simulink model "verification"  (R2012b)
settings: Solver=FixedStepDiscrete  StartTime=0.0  StopTime=10.0  FixedStep=0.1  RelTol=1e-3
undefined symbols (not defined in the file): sldvsubsys
libraries: sldvlib x21
settings Model: Creator=z2akhtar  LastModifiedBy=z2akhtar
settings ConfigComp: Description=Design Verifier Custom Configuration Component  DVMode=PropertyProving  DVMaxProcessTime=1800  DVMaxTestCaseSteps=500  DVTestSuiteOptimization=CombinedObjectives (Nonlinear Extended)  DVProvingStrategy=ProveWithViolationDetection  DVMaxViolationSteps=10

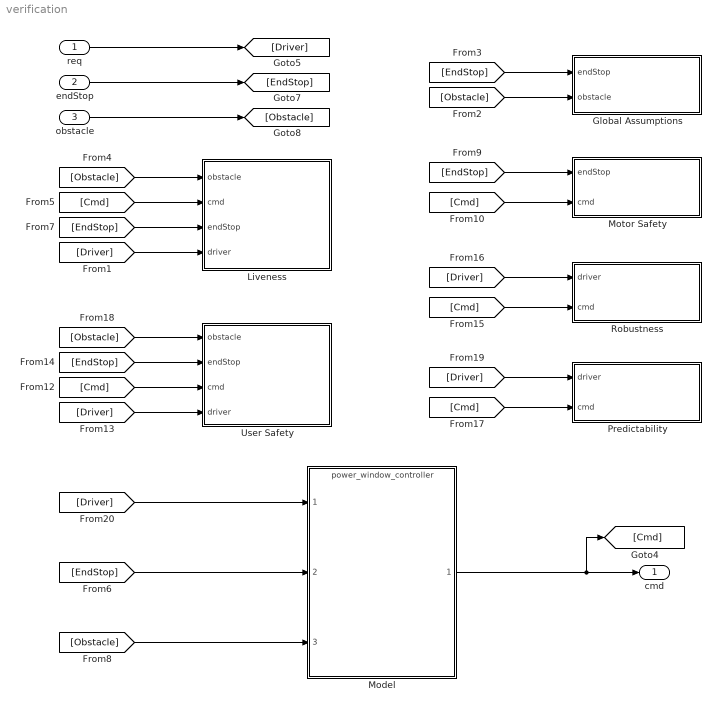
== system verification ==
  req : Inport  OutDataTypeStr=double
  endStop : Inport  Port=2  OutDataTypeStr=boolean
  obstacle : Inport  Port=3  OutDataTypeStr=boolean
  Global Assumptions : Subsystem  Tag=VerificationSubsystem  DisableCoverage=on  LoadFcn=sldvsubsys('check')  TreatAsAtomicUnit=on  SimViewingDevice=on  mask(VerificationSubsystem){}
      mask init:
      | sldvsubsys('maskInit');
      settings: CopyFcn=sldvsubsys('copy');  OpenFcn=open_system(gcb,'force');
      settings: PreSaveFcn=|
      | set_param(gcb,'SimViewingDevice','on');
      | sldvsubsys('check');
      mask Help: helpview(fullfile(docroot,'toolbox','sldv','sldv.map'),'verificationsubsystem')
      mask Display: image(imread('sldvicon_versubsys.png','BackGroundColor',[1 1 1]),'center');
  Liveness : Subsystem  Tag=VerificationSubsystem  DisableCoverage=on  LoadFcn=sldvsubsys('check')  TreatAsAtomicUnit=on  SimViewingDevice=on  mask(VerificationSubsystem){}
      mask init:
      | sldvsubsys('maskInit');
      settings: CopyFcn=sldvsubsys('copy');  OpenFcn=open_system(gcb,'force');
      settings: PreSaveFcn=|
      | set_param(gcb,'SimViewingDevice','on');
      | sldvsubsys('check');
      mask Help: helpview(fullfile(docroot,'toolbox','sldv','sldv.map'),'verificationsubsystem')
      mask Display: image(imread('sldvicon_versubsys.png','BackGroundColor',[1 1 1]),'center');
  Model : ModelReference  ModelNameDialog=power_window_controller  SimulationMode=Normal  ModelReferenceVersion=1.36  CopyOfModelName=power_window_controller  DefaultDataLogging=on
  Motor Safety : Subsystem  Tag=VerificationSubsystem  DisableCoverage=on  LoadFcn=sldvsubsys('check')  TreatAsAtomicUnit=on  SimViewingDevice=on  mask(VerificationSubsystem){}
      mask init:
      | sldvsubsys('maskInit');
      settings: CopyFcn=sldvsubsys('copy');  OpenFcn=open_system(gcb,'force');
      settings: PreSaveFcn=|
      | set_param(gcb,'SimViewingDevice','on');
      | sldvsubsys('check');
      mask Help: helpview(fullfile(docroot,'toolbox','sldv','sldv.map'),'verificationsubsystem')
      mask Display: image(imread('sldvicon_versubsys.png','BackGroundColor',[1 1 1]),'center');
  Predictability : Subsystem  Tag=VerificationSubsystem  DisableCoverage=on  LoadFcn=sldvsubsys('check')  TreatAsAtomicUnit=on  SimViewingDevice=on  mask(VerificationSubsystem){}
      mask init:
      | sldvsubsys('maskInit');
      settings: CopyFcn=sldvsubsys('copy');  OpenFcn=open_system(gcb,'force');
      settings: PreSaveFcn=|
      | set_param(gcb,'SimViewingDevice','on');
      | sldvsubsys('check');
      mask Help: helpview(fullfile(docroot,'toolbox','sldv','sldv.map'),'verificationsubsystem')
      mask Display: image(imread('sldvicon_versubsys.png','BackGroundColor',[1 1 1]),'center');
  Robustness : Subsystem  Tag=VerificationSubsystem  DisableCoverage=on  LoadFcn=sldvsubsys('check')  TreatAsAtomicUnit=on  SimViewingDevice=on  mask(VerificationSubsystem){}
      mask init:
      | sldvsubsys('maskInit');
      settings: CopyFcn=sldvsubsys('copy');  OpenFcn=open_system(gcb,'force');
      settings: PreSaveFcn=|
      | set_param(gcb,'SimViewingDevice','on');
      | sldvsubsys('check');
      mask Help: helpview(fullfile(docroot,'toolbox','sldv','sldv.map'),'verificationsubsystem')
      mask Display: image(imread('sldvicon_versubsys.png','BackGroundColor',[1 1 1]),'center');
  User Safety : Subsystem  Tag=VerificationSubsystem  DisableCoverage=on  LoadFcn=sldvsubsys('check')  TreatAsAtomicUnit=on  SimViewingDevice=on  mask(VerificationSubsystem){}
      mask init:
      | sldvsubsys('maskInit');
      settings: CopyFcn=sldvsubsys('copy');  OpenFcn=open_system(gcb,'force');
      settings: PreSaveFcn=|
      | set_param(gcb,'SimViewingDevice','on');
      | sldvsubsys('check');
      mask Help: helpview(fullfile(docroot,'toolbox','sldv','sldv.map'),'verificationsubsystem')
      mask Display: image(imread('sldvicon_versubsys.png','BackGroundColor',[1 1 1]),'center');
  cmd : Outport
  wires:
  Model/1 -> [Cmd], cmd/1
  req/1 -> [Driver]
  endStop/1 -> [EndStop]
  obstacle/1 -> [Obstacle]
  [Obstacle] -> Global Assumptions/2(obstacle)
  [EndStop] -> Global Assumptions/1(endStop)
  [EndStop] -> Motor Safety/1(endStop)
  [Cmd] -> Motor Safety/2(cmd)
  [EndStop] -> User Safety/2(endStop)
  [Cmd] -> User Safety/3(cmd)
  [Driver] -> User Safety/4(driver)
  [Driver] -> Model/1
  [EndStop] -> Model/2
  [Obstacle] -> Model/3
  [Cmd] -> Robustness/2(cmd)
  [Driver] -> Robustness/1(driver)
  [Obstacle] -> User Safety/1(obstacle)
  [Obstacle] -> Liveness/1(obstacle)
  [Cmd] -> Liveness/2(cmd)
  [EndStop] -> Liveness/3(endStop)
  [Driver] -> Liveness/4(driver)
  [Cmd] -> Predictability/2(cmd)
  [Driver] -> Predictability/1(driver)

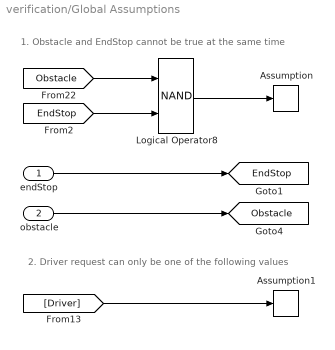
== system verification/Global Assumptions ==
  note: 1. Obstacle and EndStop cannot be true at the same time
  note: 2. Driver request can only be one of the following values
  endStop : Inport
  obstacle : Inport  Port=2
  Assumption : sldvlib/Objectives and Constraints/Assumption  enabled=on  customAVTBlockType=Assumption  intervals=true  initial=off  dispValues=on  outEnabled=off
      settings: AttributesFormatString=%<intervals>
  Assumption1 : sldvlib/Objectives and Constraints/Assumption  enabled=on  customAVTBlockType=Assumption  intervals={0,1,2,3,4}  initial=off  dispValues=on  outEnabled=off
      settings: AttributesFormatString=%<intervals>
  Logical Operator8 : Logic  Operator=NAND  AllPortsSameDT=off  OutDataTypeStr=boolean
  tag scope: EndStop=global, Obstacle=global
  wires:
  [Obstacle] -> Logical Operator8/1
  Logical Operator8/1 -> Assumption/1
  [EndStop] -> Logical Operator8/2
  endStop/1 -> [EndStop]
  obstacle/1 -> [Obstacle]
  [Driver] -> Assumption1/1

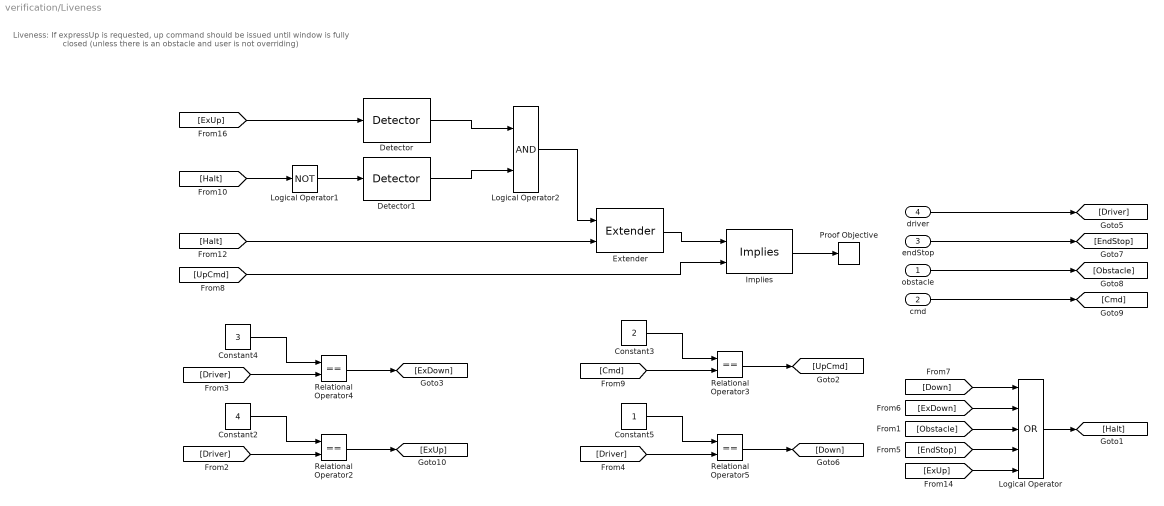
== system verification/Liveness ==
  note: Liveness:
      | If expressUp is requested, up command should be issued until window is fully closed (unless there is an obstacle and user is not overriding)
  obstacle : Inport  OutDataTypeStr=boolean
  cmd : Inport  Port=2
  endStop : Inport  Port=3  OutDataTypeStr=boolean
  driver : Inport  Port=4  OutDataTypeStr=double
  Constant2 : Constant  Value=4  SampleTime=Inf
  Constant3 : Constant  Value=2  SampleTime=Inf
  Constant4 : Constant  Value=3  SampleTime=Inf
  Constant5 : Constant  SampleTime=Inf
  Detector : sldvlib/Temporal Operators/Detector  reset=off  typ=Delayed Fixed Duration  in_hold=3  delay=0  out_hold=2
  Detector1 : sldvlib/Temporal Operators/Detector  reset=off  typ=Delayed Fixed Duration  in_hold=4  delay=0  out_hold=1
  Extender : sldvlib/Temporal Operators/Extender  reset=on  ext_type=Infinite  out_hold=3
  Implies : sldvlib/Verification Utilities/Implies
  Logical Operator : Logic  Operator=OR  Inputs=5  AllPortsSameDT=off  OutDataTypeStr=boolean
  Logical Operator1 : Logic  Operator=NOT  AllPortsSameDT=off  OutDataTypeStr=boolean
  Logical Operator2 : Logic  AllPortsSameDT=off  OutDataTypeStr=boolean
  Proof Objective : sldvlib/Objectives and Constraints/Proof Objective  enabled=on  customAVTBlockType=Proof Objective  intervals=true  dispValues=on  outEnabled=off  enableStopSim=off
      settings: AttributesFormatString=%<intervals>
  Relational Operator{2..5} (4 alike) : RelationalOperator  Operator===  OutDataTypeStr=boolean
  wires:
  Implies/1 -> Proof Objective/1
  [Driver] -> Relational Operator2/2
  Constant2/1 -> Relational Operator2/1
  Relational Operator2/1 -> [ExUp]
  [ExUp] -> Detector/1
  [Cmd] -> Relational Operator3/2
  Constant3/1 -> Relational Operator3/1
  Relational Operator3/1 -> [UpCmd]
  driver/1 -> [Driver]
  endStop/1 -> [EndStop]
  obstacle/1 -> [Obstacle]
  [Driver] -> Relational Operator4/2
  Constant4/1 -> Relational Operator4/1
  Relational Operator4/1 -> [ExDown]
  [Driver] -> Relational Operator5/2
  Constant5/1 -> Relational Operator5/1
  Relational Operator5/1 -> [Down]
  Logical Operator/1 -> [Halt]
  [Down] -> Logical Operator/1
  [ExDown] -> Logical Operator/2
  [Obstacle] -> Logical Operator/3
  [EndStop] -> Logical Operator/4
  cmd/1 -> [Cmd]
  [Halt] -> Logical Operator1/1
  Logical Operator2/1 -> Extender/1
  [Halt] -> Extender/2
  [UpCmd] -> Implies/2
  Extender/1 -> Implies/1
  Detector/1 -> Logical Operator2/1
  Logical Operator1/1 -> Detector1/1
  Detector1/1 -> Logical Operator2/2
  [ExUp] -> Logical Operator/5

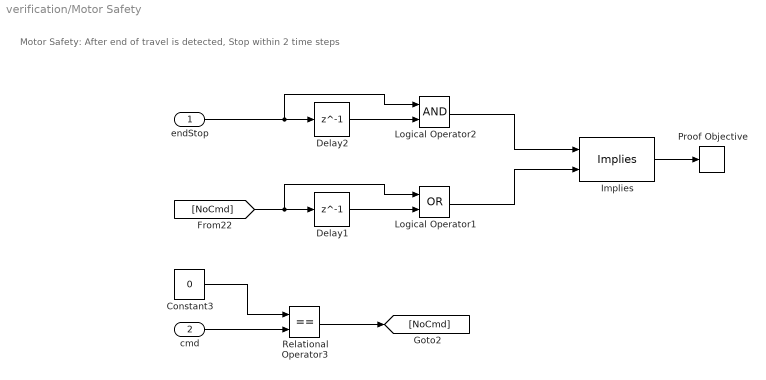
== system verification/Motor Safety ==
  note: Motor Safety:
      | After end of travel is detected, Stop within 2 time steps
  endStop : Inport
  cmd : Inport  Port=2
  Constant3 : Constant  Value=0  SampleTime=Inf
  Delay1 : Delay  DelayLength=1  InitialCondition=0
  Delay2 : Delay  DelayLength=1  InitialCondition=0
  Implies : sldvlib/Verification Utilities/Implies
  Logical Operator1 : Logic  Operator=OR  AllPortsSameDT=off  OutDataTypeStr=boolean
  Logical Operator2 : Logic  AllPortsSameDT=off  OutDataTypeStr=boolean
  Proof Objective : sldvlib/Objectives and Constraints/Proof Objective  enabled=off  customAVTBlockType=Proof Objective  intervals=true  dispValues=on  outEnabled=off  enableStopSim=off
      settings: AttributesFormatString=%<intervals>
  Relational Operator3 : RelationalOperator  Operator===  OutDataTypeStr=boolean
  wires:
  Implies/1 -> Proof Objective/1
  Delay1/1 -> Logical Operator1/2
  [NoCmd] -> Delay1/1, Logical Operator1/1
  cmd/1 -> Relational Operator3/2
  Constant3/1 -> Relational Operator3/1
  Relational Operator3/1 -> [NoCmd]
  Delay2/1 -> Logical Operator2/2
  endStop/1 -> Delay2/1, Logical Operator2/1
  Logical Operator2/1 -> Implies/1
  Logical Operator1/1 -> Implies/2

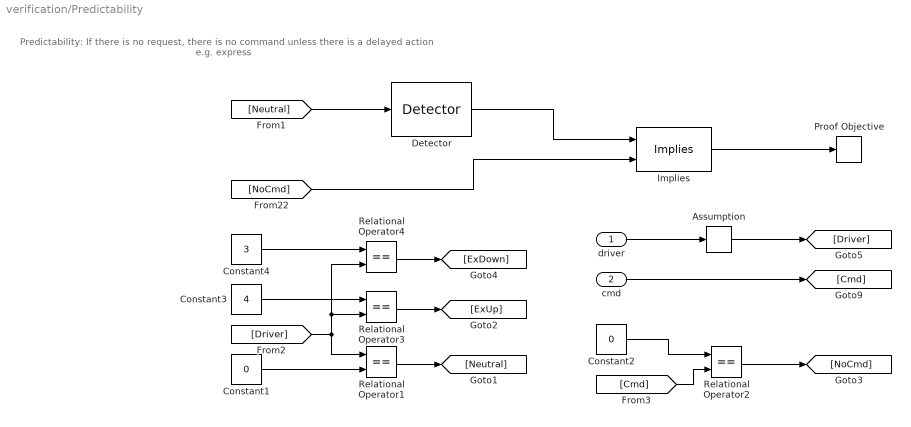
== system verification/Predictability ==
  note: Predictability:
      | If there is no request, there is no command unless there is a delayed action e.g. express
  driver : Inport  OutDataTypeStr=double
  cmd : Inport  Port=2
  Assumption : sldvlib/Objectives and Constraints/Assumption  enabled=on  customAVTBlockType=Assumption  intervals={0,1,2}  initial=off  dispValues=on  outEnabled=on
      settings: AttributesFormatString=%<intervals>
  Constant1 : Constant  Value=0  SampleTime=Inf
  Constant2 : Constant  Value=0  SampleTime=Inf
  Constant3 : Constant  Value=4  SampleTime=Inf
  Constant4 : Constant  Value=3  SampleTime=Inf
  Detector : sldvlib/Temporal Operators/Detector  reset=off  typ=Synchronized  in_hold=3  delay=0  out_hold=5
  Implies : sldvlib/Verification Utilities/Implies
  Proof Objective : sldvlib/Objectives and Constraints/Proof Objective  enabled=on  customAVTBlockType=Proof Objective  intervals=true  dispValues=on  outEnabled=off  enableStopSim=off
      settings: AttributesFormatString=%<intervals>
  Relational Operator{1..4} (4 alike) : RelationalOperator  Operator===  OutDataTypeStr=boolean
  wires:
  Implies/1 -> Proof Objective/1
  [Driver] -> Relational Operator4/2, Relational Operator3/2, Relational Operator1/1
  Relational Operator3/1 -> [ExUp]
  Constant1/1 -> Relational Operator1/2
  Constant3/1 -> Relational Operator3/1
  Relational Operator1/1 -> [Neutral]
  [Neutral] -> Detector/1
  Relational Operator2/1 -> [NoCmd]
  cmd/1 -> [Cmd]
  Constant4/1 -> Relational Operator4/1
  Relational Operator4/1 -> [ExDown]
  driver/1 -> Assumption/1
  Assumption/1 -> [Driver]
  Detector/1 -> Implies/1
  [Cmd] -> Relational Operator2/2
  Constant2/1 -> Relational Operator2/1
  [NoCmd] -> Implies/2

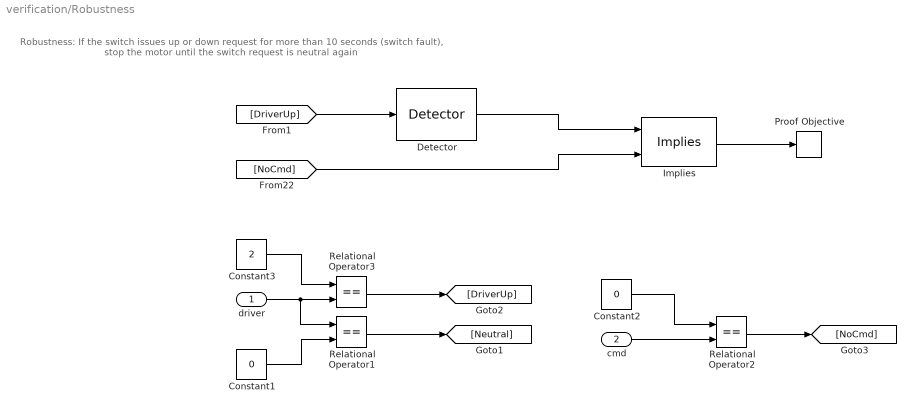
== system verification/Robustness ==
  note: Robustness:
      | If the switch issues up or down request for more than 10 seconds (switch fault), stop the motor until the switch request is neutral again
  driver : Inport
  cmd : Inport  Port=2
  Constant1 : Constant  Value=0  SampleTime=Inf
  Constant2 : Constant  Value=0  SampleTime=Inf
  Constant3 : Constant  Value=2  SampleTime=Inf
  Detector : sldvlib/Temporal Operators/Detector  reset=off  typ=Delayed Fixed Duration  in_hold=100  delay=0  out_hold=5
  Implies : sldvlib/Verification Utilities/Implies
  Proof Objective : sldvlib/Objectives and Constraints/Proof Objective  enabled=off  customAVTBlockType=Proof Objective  intervals=true  dispValues=on  outEnabled=off  enableStopSim=off
      settings: AttributesFormatString=%<intervals>
  Relational Operator1 : RelationalOperator  Operator===  OutDataTypeStr=boolean
  Relational Operator2 : RelationalOperator  Operator===  OutDataTypeStr=boolean
  Relational Operator3 : RelationalOperator  Operator===  OutDataTypeStr=boolean
  wires:
  Implies/1 -> Proof Objective/1
  driver/1 -> Relational Operator1/1, Relational Operator3/2
  Relational Operator3/1 -> [DriverUp]
  [NoCmd] -> Implies/2
  Constant1/1 -> Relational Operator1/2
  Constant3/1 -> Relational Operator3/1
  Relational Operator1/1 -> [Neutral]
  [DriverUp] -> Detector/1
  Detector/1 -> Implies/1
  cmd/1 -> Relational Operator2/2
  Constant2/1 -> Relational Operator2/1
  Relational Operator2/1 -> [NoCmd]

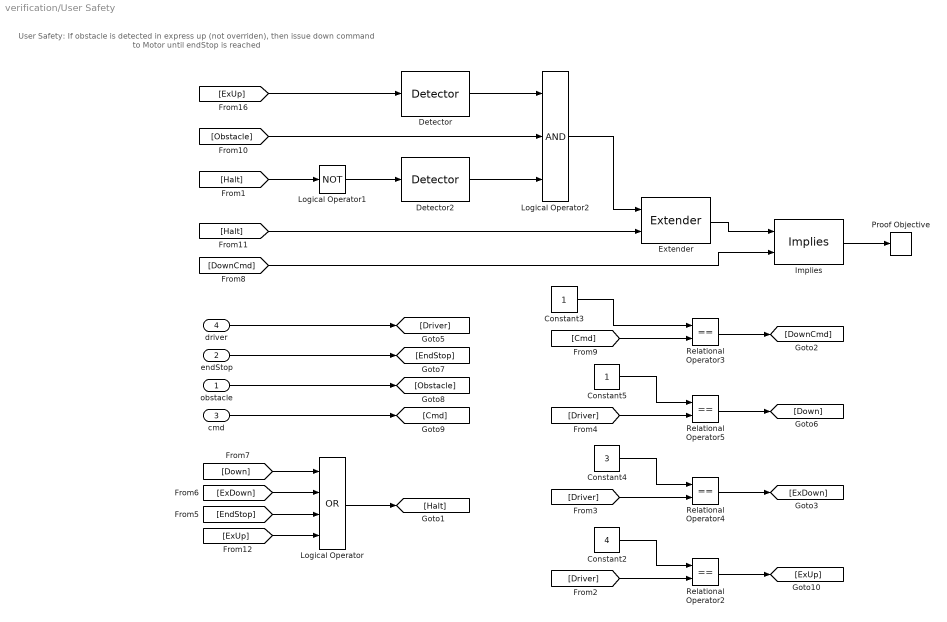
== system verification/User Safety ==
  note: User Safety:
      | If obstacle is detected in express up (not overriden), then issue down command to Motor until endStop is reached
  obstacle : Inport  OutDataTypeStr=boolean
  endStop : Inport  Port=2  OutDataTypeStr=boolean
  cmd : Inport  Port=3
  driver : Inport  Port=4  OutDataTypeStr=double
  Constant2 : Constant  Value=4  SampleTime=Inf
  Constant3 : Constant  SampleTime=Inf
  Constant4 : Constant  Value=3  SampleTime=Inf
  Constant5 : Constant  SampleTime=Inf
  Detector : sldvlib/Temporal Operators/Detector  reset=off  typ=Delayed Fixed Duration  in_hold=3  delay=0  out_hold=2
  Detector2 : sldvlib/Temporal Operators/Detector  reset=off  typ=Delayed Fixed Duration  in_hold=4  delay=0  out_hold=1
  Extender : sldvlib/Temporal Operators/Extender  reset=on  ext_type=Infinite  out_hold=3
  Implies : sldvlib/Verification Utilities/Implies
  Logical Operator : Logic  Operator=OR  Inputs=4  AllPortsSameDT=off  OutDataTypeStr=boolean
  Logical Operator1 : Logic  Operator=NOT  AllPortsSameDT=off  OutDataTypeStr=boolean
  Logical Operator2 : Logic  Inputs=3  AllPortsSameDT=off  OutDataTypeStr=boolean
  Proof Objective : sldvlib/Objectives and Constraints/Proof Objective  enabled=on  customAVTBlockType=Proof Objective  intervals=true  dispValues=on  outEnabled=off  enableStopSim=off
      settings: AttributesFormatString=%<intervals>
  Relational Operator{2..5} (4 alike) : RelationalOperator  Operator===  OutDataTypeStr=boolean
  wires:
  Implies/1 -> Proof Objective/1
  [Driver] -> Relational Operator2/2
  Constant2/1 -> Relational Operator2/1
  Relational Operator2/1 -> [ExUp]
  [ExUp] -> Detector/1
  [Cmd] -> Relational Operator3/2
  Constant3/1 -> Relational Operator3/1
  Relational Operator3/1 -> [DownCmd]
  driver/1 -> [Driver]
  endStop/1 -> [EndStop]
  obstacle/1 -> [Obstacle]
  [Driver] -> Relational Operator4/2
  Constant4/1 -> Relational Operator4/1
  Relational Operator4/1 -> [ExDown]
  [Driver] -> Relational Operator5/2
  Constant5/1 -> Relational Operator5/1
  Relational Operator5/1 -> [Down]
  Logical Operator/1 -> [Halt]
  [Down] -> Logical Operator/1
  [ExDown] -> Logical Operator/2
  cmd/1 -> [Cmd]
  Logical Operator2/1 -> Extender/1
  [Halt] -> Extender/2
  [DownCmd] -> Implies/2
  Extender/1 -> Implies/1
  Detector2/1 -> Logical Operator2/3
  [Obstacle] -> Logical Operator2/2
  Logical Operator1/1 -> Detector2/1
  [Halt] -> Logical Operator1/1
  Detector/1 -> Logical Operator2/1
  [EndStop] -> Logical Operator/3
  [ExUp] -> Logical Operator/4
